simulink model "lastfuzzy"  (Simulink 5.0)
settings: Solver=ode5  StartTime=0.0  StopTime=50  FixedStep=0.001  RelTol=1e-3
InitFcn:
  | init_para
undefined symbols (not defined in the file): a, dzcv, fc, fp, fs, g, j, l, M, mi, u1, u2, xc, yc
libraries: simulink x2
settings Model: LastModifiedBy=AD

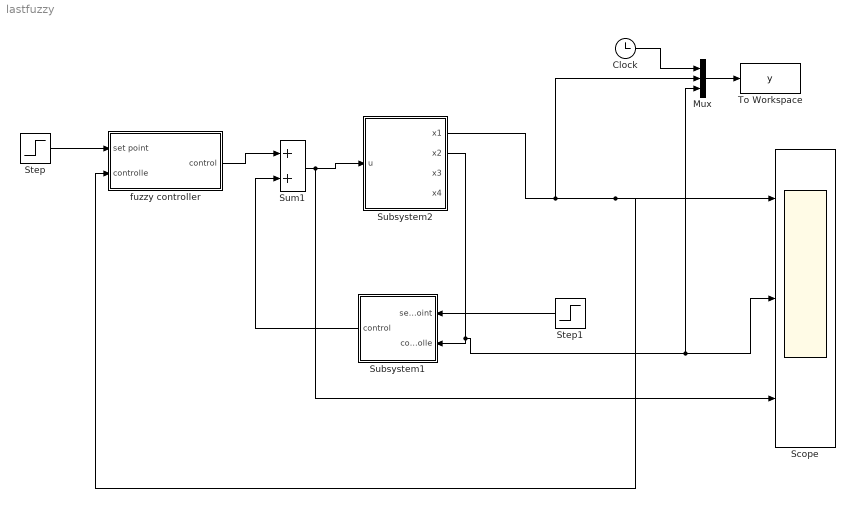
== system lastfuzzy ==
  Clock : Clock
      settings: Decimation=10
  Mux : Mux  Inputs=3
  Scope : Scope  NumInputPorts=3
      settings: TimeRange=50  YMin=-5~-5~-5  YMax=5~5~5
  Step : Step  Time=20  Before=pi  After=0.2  SampleTime=0
  Step1 : Step  Orientation=left  Time=0  Before=pi  After=0  SampleTime=0
  Subsystem1 : Subsystem  Orientation=left
  Subsystem2 : Subsystem
  Sum1 : Sum  SaturateOnIntegerOverflow=on
  To Workspace : ToWorkspace  VariableName=y  SampleTime=-1  SaveFormat=Array
  fuzzy controller : Subsystem
  wires:
  Step/1 -> fuzzy controller/1(set point)
  fuzzy controller/1(control) -> Sum1/1
  Subsystem1/1(control) -> Sum1/2
  Step1/1 -> Subsystem1/1(set point)
  Sum1/1 -> Subsystem2/1(u), Scope/3
  Subsystem2/1(x1) -> Scope/1, fuzzy controller/2(controlle), Mux/2
  Subsystem2/2(x2) -> Subsystem1/2(controlle), Scope/2, Mux/3
  Clock/1 -> Mux/1
  Mux/1 -> To Workspace/1

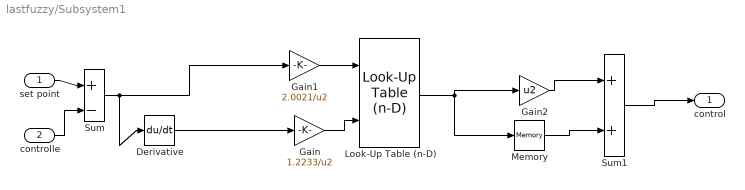
== system lastfuzzy/Subsystem1 ==
  set point : Inport
  controlle : Inport  Port=2
  Derivative : Derivative
  Gain : Gain  Gain=1.2233/u2  SaturateOnIntegerOverflow=on
  Gain1 : Gain  Gain=2.0021/u2  SaturateOnIntegerOverflow=on
  Gain2 : Gain  Gain=u2  SaturateOnIntegerOverflow=on
  Look-Up Table (n-D) : simulink/Look-Up Tables/Look-Up Table (n-D)  numDimsPopupSelect=2  bp1=-2:.05:2  bp2=-2:.05:2  bp3=[1:3]  bp4=[1:3]  bpcell={ [1:3], [1:3] }  explicitNumDims=2  searchMode=Binary Search  cacheBpFlag=off  vectorInputFlag=off  tableData=P  interpMethod=Linear  extrapMethod=Linear  rangeErrorMode=None
  Memory : Memory  InheritSampleTime=on
  Sum : Sum  Inputs=|+-  SaturateOnIntegerOverflow=on
  Sum1 : Sum  SaturateOnIntegerOverflow=on
  control : Outport
  wires:
  Sum1/1 -> control/1
  Gain2/1 -> Sum1/1
  Look-Up Table (n-D)/1 -> Memory/1, Gain2/1
  controlle/1 -> Sum/2
  set point/1 -> Sum/1
  Sum/1 -> Derivative/1, Gain1/1
  Gain/1 -> Look-Up Table (n-D)/2
  Gain1/1 -> Look-Up Table (n-D)/1
  Derivative/1 -> Gain/1
  Memory/1 -> Sum1/2

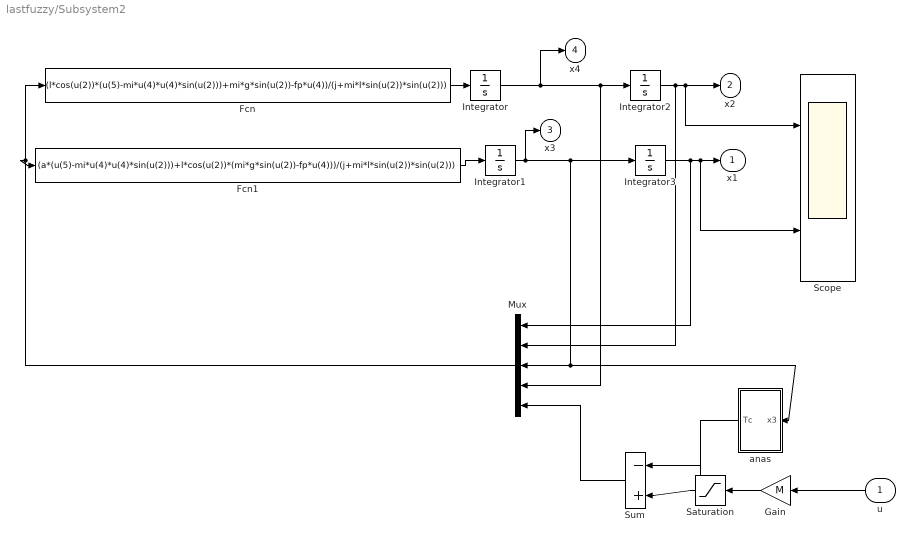
== system lastfuzzy/Subsystem2 ==
  u : Inport  Orientation=left
  Fcn : Fcn  Expr=(l*cos(u(2))*(u(5)-mi*u(4)*u(4)*sin(u(2)))+mi*g*sin(u(2))-fp*u(4))/(j+mi*l*sin(u(2))*sin(u(2)))
  Fcn1 : Fcn  Expr=(a*(u(5)-mi*u(4)*u(4)*sin(u(2)))+l*cos(u(2))*(mi*g*sin(u(2))-fp*u(4)))/(j+mi*l*sin(u(2))*sin(u(2)))
  Gain : Gain  Orientation=left  Gain=M  SaturateOnIntegerOverflow=on
  Integrator{,1..3} (4 alike) : Integrator
  Mux : Mux  Orientation=left  Inputs=5
  Saturation : Saturate  Orientation=left  UpperLimit=17  LowerLimit=-17
  Scope : Scope  NumInputPorts=2
      settings: YMin=-5~-5  YMax=5~5
  Sum : Sum  Orientation=left  Inputs=|-+  SaturateOnIntegerOverflow=on
  anas : Subsystem  Orientation=left
  x1 : Outport
  x2 : Outport  Port=2
  x3 : Outport  Port=3
  x4 : Outport  Port=4
  wires:
  Fcn/1 -> Integrator/1
  Fcn1/1 -> Integrator1/1
  Integrator/1 -> Integrator2/1, Mux/4, x4/1
  Integrator1/1 -> Integrator3/1, Mux/3, anas/1(x3), x3/1
  Integrator2/1 -> Mux/2, x2/1, Scope/1
  Integrator3/1 -> Mux/1, x1/1, Scope/2
  Mux/1 -> Fcn1/1, Fcn/1
  Sum/1 -> Mux/5
  Gain/1 -> Saturation/1
  Saturation/1 -> Sum/2
  u/1 -> Gain/1
  anas/1(Tc) -> Sum/1

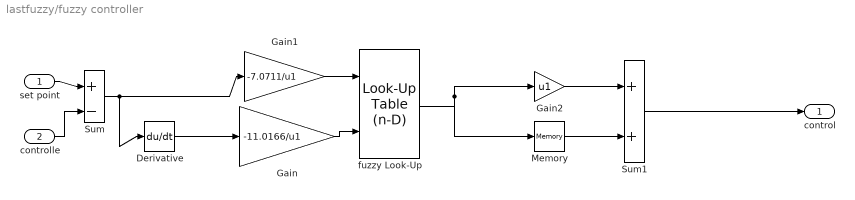
== system lastfuzzy/fuzzy controller ==
  set point : Inport
  controlle : Inport  Port=2
  Derivative : Derivative
  Gain : Gain  Gain=-11.0166/u1  SaturateOnIntegerOverflow=on
  Gain1 : Gain  Gain=-7.0711/u1  SaturateOnIntegerOverflow=on
  Gain2 : Gain  Gain=u1  SaturateOnIntegerOverflow=on
  Memory : Memory  InheritSampleTime=on
  Sum : Sum  Inputs=|+-  SaturateOnIntegerOverflow=on
  Sum1 : Sum  SaturateOnIntegerOverflow=on
  "fuzzy Look-Up " : simulink/Look-Up Tables/Look-Up Table (n-D)  numDimsPopupSelect=2  bp1=-2:.05:2  bp2=-2:.05:2  bp3=[1:3]  bp4=[1:3]  bpcell={ [1:3], [1:3] }  explicitNumDims=2  searchMode=Binary Search  cacheBpFlag=off  vectorInputFlag=off  tableData=P  interpMethod=Linear  extrapMethod=Linear  rangeErrorMode=None
  control : Outport
  wires:
  Derivative/1 -> Gain/1
  Gain1/1 -> "fuzzy Look-Up "/1
  Gain/1 -> "fuzzy Look-Up "/2
  Sum/1 -> Gain1/1, Derivative/1
  set point/1 -> Sum/1
  controlle/1 -> Sum/2
  "fuzzy Look-Up "/1 -> Gain2/1, Memory/1
  Gain2/1 -> Sum1/1
  Sum1/1 -> control/1
  Memory/1 -> Sum1/2

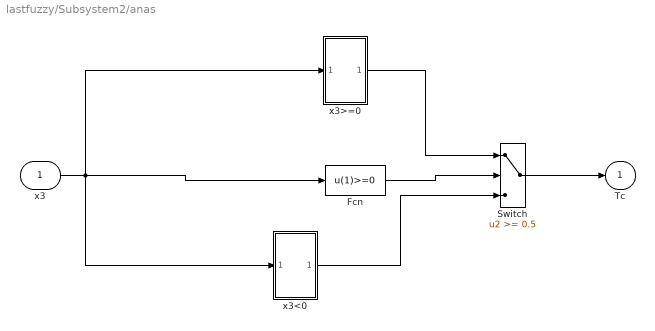
== system lastfuzzy/Subsystem2/anas ==
  x3 : Inport
  Fcn : Fcn  Expr=u(1)>=0
  Switch : Switch  Threshold=0.5  SaturateOnIntegerOverflow=on
  x3<0 : Subsystem
  x3>=0 : Subsystem
  Tc : Outport
  wires:
  Switch/1 -> Tc/1
  Fcn/1 -> Switch/2
  x3/1 -> Fcn/1, x3>=0/1(In1), x3<0/1(In1)
  x3>=0/1(out1) -> Switch/1
  x3<0/1(out1) -> Switch/3

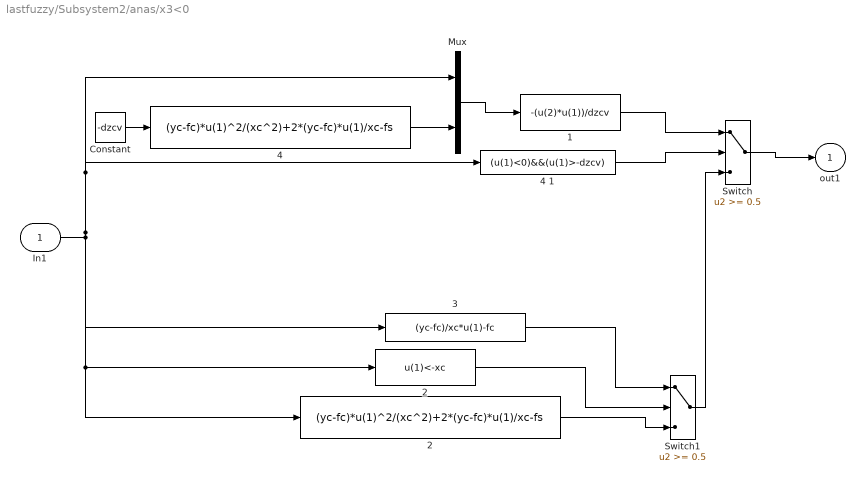
== system lastfuzzy/Subsystem2/anas/x3<0 ==
  In1 : Inport
  1 : Fcn  Expr=-(u(2)*u(1))/dzcv
  2 : Fcn  Expr=u(1)<-xc
  "2 " : Fcn  Expr=(yc-fc)*u(1)^2/(xc^2)+2*(yc-fc)*u(1)/xc-fs
  3 : Fcn  Expr=(yc-fc)/xc*u(1)-fc
  "4 " : Fcn  Expr=(yc-fc)*u(1)^2/(xc^2)+2*(yc-fc)*u(1)/xc-fs
  4 1 : Fcn  Expr=(u(1)<0)&&(u(1)>-dzcv)
  Constant : Constant  Value=-dzcv
  Mux : Mux  Inputs=2
  Switch : Switch  Threshold=0.5  SaturateOnIntegerOverflow=on
  Switch1 : Switch  Threshold=0.5  SaturateOnIntegerOverflow=on
  out1 : Outport
  wires:
  1/1 -> Switch/1
  3/1 -> Switch1/1
  2/1 -> Switch1/2
  "2 "/1 -> Switch1/3
  Switch1/1 -> Switch/3
  Mux/1 -> 1/1
  "4 "/1 -> Mux/2
  In1/1 -> 3/1, 2/1, "2 "/1, Mux/1, 4 1/1
  Constant/1 -> "4 "/1
  4 1/1 -> Switch/2
  Switch/1 -> out1/1

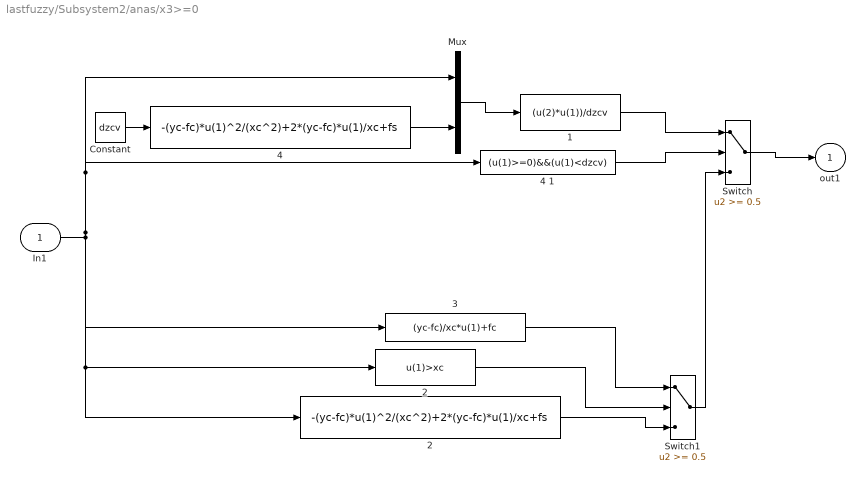
== system lastfuzzy/Subsystem2/anas/x3>=0 ==
  In1 : Inport
  1 : Fcn  Expr=(u(2)*u(1))/dzcv
  2 : Fcn  Expr=u(1)>xc
  "2 " : Fcn  Expr=-(yc-fc)*u(1)^2/(xc^2)+2*(yc-fc)*u(1)/xc+fs
  3 : Fcn  Expr=(yc-fc)/xc*u(1)+fc
  "4 " : Fcn  Expr=-(yc-fc)*u(1)^2/(xc^2)+2*(yc-fc)*u(1)/xc+fs
  4 1 : Fcn  Expr=(u(1)>=0)&&(u(1)<dzcv)
  Constant : Constant  Value=dzcv
  Mux : Mux  Inputs=2
  Switch : Switch  Threshold=0.5  SaturateOnIntegerOverflow=on
  Switch1 : Switch  Threshold=0.5  SaturateOnIntegerOverflow=on
  out1 : Outport
  wires:
  1/1 -> Switch/1
  3/1 -> Switch1/1
  2/1 -> Switch1/2
  "2 "/1 -> Switch1/3
  Switch1/1 -> Switch/3
  Mux/1 -> 1/1
  "4 "/1 -> Mux/2
  In1/1 -> 3/1, 2/1, "2 "/1, Mux/1, 4 1/1
  Constant/1 -> "4 "/1
  4 1/1 -> Switch/2
  Switch/1 -> out1/1
